simulink model "electromagnet_c"  (R2024a)
settings: Solver=VariableStepAuto  StartTime=0.0  StopTime=te  MaxStep=te/100  RelTol=1e-3
values from neighbouring files (symbols this model uses):
  A = 9e-4    (= 0.0009)    [Electromagnet_par.m]    (also in coil_ironcore.m = 0.0005; sim21_ODE.m = 2)
  lfe = 0.15    [Electromagnet_par.m]
  mu0 = 4e-7*pi    (= 1.25663706144e-06)    [Electromagnet_par.m]    (also in coil_ironcore.m)
  mur = 200    [Electromagnet_par.m]    (also in coil_ironcore.m = 1000)
  N = 900    [Electromagnet_par.m]    (also in coil_ironcore.m = 1000)
  R = 6.5    [Electromagnet_par.m]    (also in coil_ironcore.m = 10; sim21_ODE.m = 10)
  U = 10    [Electromagnet_par.m]    (also in coil_ironcore.m = 163; sim21_ODE.m = 230*sqrt(2))
  w = 2*pi/0.1    (= 62.8318530718)    [Electromagnet_par.m]    (also in coil_ironcore.m = 314.159265359; sim21_ODE.m = [0.5 1 2])
  x0 = 0.01    [Electromagnet_par.m]    (also in sim21_ODE.m = [0 0])
settings Model: Creator=ocean  LastModifiedBy=ocean

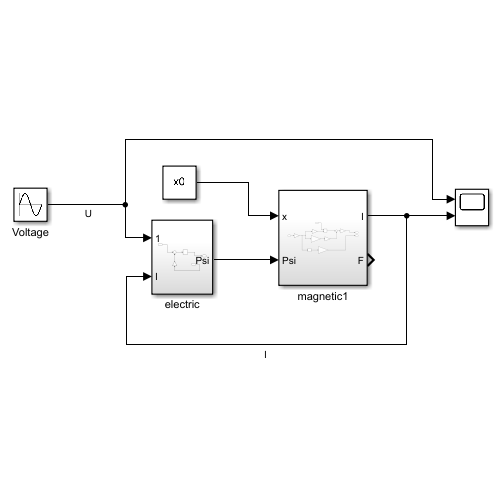
[thumbnail: Simulink's stored preview of the top-level diagram]
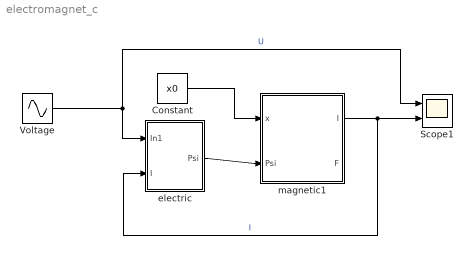
== system electromagnet_c ==
  Constant : Constant  Value=x0
  Scope1 : Scope  NumInputPorts=2
  Voltage : Sin  Amplitude=U  Frequency=w  SampleTime=0
  electric : Subsystem
  magnetic1 : Subsystem
  wires:
  Voltage/1 -> electric/1(In1), Scope1/1  "U"
  magnetic1/1(I) -> Scope1/2, electric/2(I)  "I"
  electric/1(Psi) -> magnetic1/2(Psi)
  Constant/1 -> magnetic1/1(x)

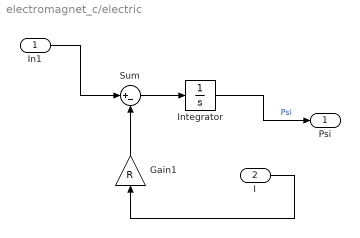
== system electromagnet_c/electric ==
  In1 : Inport
  I : Inport  Port=2
  Gain1 : Gain  Gain=R
  Integrator : Integrator
  Sum : Sum  Inputs=|+-
  Psi : Outport
  wires:
  Gain1/1 -> Sum/2
  Sum/1 -> Integrator/1
  I/1 -> Gain1/1
  In1/1 -> Sum/1
  Integrator/1 -> Psi/1  "Psi"

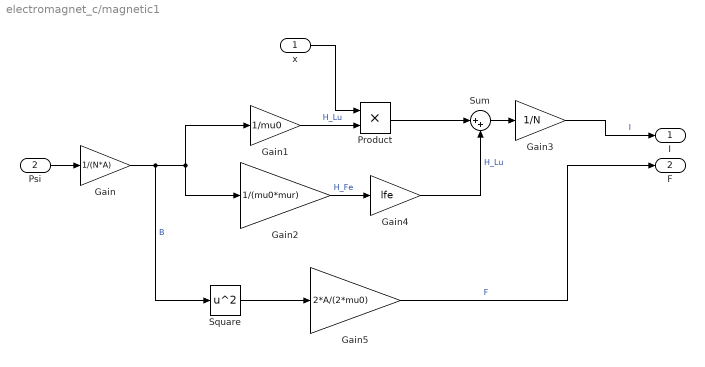
== system electromagnet_c/magnetic1 ==
  x : Inport
  Psi : Inport  Port=2
  Gain : Gain  Gain=1/(N*A)
  Gain1 : Gain  Gain=1/mu0
  Gain2 : Gain  Gain=1/(mu0*mur)
  Gain3 : Gain  Gain=1/N
  Gain4 : Gain  Gain=lfe
  Gain5 : Gain  Gain=2*A/(2*mu0)
  Product : Product
  Square : Math  Operator=square
  Sum : Sum  Inputs=|++
  I : Outport
  F : Outport  Port=2
  wires:
  Product/1 -> Sum/1
  Square/1 -> Gain5/1
  Gain/1 -> Square/1, Gain1/1, Gain2/1  "B"
  Gain4/1 -> Sum/2  "H_Lu"
  Gain2/1 -> Gain4/1  "H_Fe"
  Gain1/1 -> Product/2  "H_Lu"
  Sum/1 -> Gain3/1
  Gain3/1 -> I/1  "I"
  x/1 -> Product/1
  Gain5/1 -> F/1  "F"
  Psi/1 -> Gain/1
